simulink model "ExampleHeadTracking"  (Simulink 9.2)
settings: Solver=FixedStepDiscrete  StartTime=0.0  StopTime=inf  FixedStep=0.001  RelTol=1e-3  EnableMultiTasking=on
libraries: rFproPhysicsLib x3
settings Model: Creator=enewton  LastModifiedBy=SeanKavanagh
settings OptimizationCC: ExpressionDepthLimit=2147483647
settings DebuggingCC: SolverPrmCheckMsg=warning
settings RTWCC: SystemTargetFile=rfpro.tlc  MakeCommand="make_rtw OPTS=\"-DRUN_PHYSICS\""  TemplateMakefile=rfpro.tmf  Description=rFpro Target (Run Physics)  TargetLang=C++
settings STFCustomTargetCC: ModelReferenceCompliant=off  GeneratePreprocessorConditionals=Disable all  CombineOutputUpdateFcns=on  MatFileLogging=on  CPPClassGenCompliant=on  GRTInterface=off  SystemTargetFile=rfpro.tlc
settings GRTTargetCC: ModelReferenceCompliant=off  ParMdlRefBuildCompliant=off  CompOptLevelCompliant=off  ConcurrentExecutionCompliant=off  CombineOutputUpdateFcns=on  GRTInterface=off  UseToolchainInfoCompliant=off

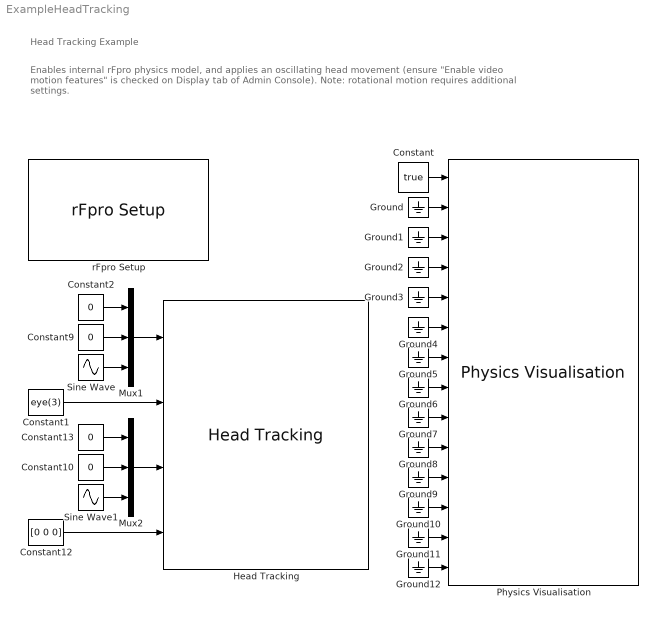
== system ExampleHeadTracking ==
  note: Enables internal rFpro physics model, and applies an oscillating head movement
      | (ensure "Enable video motion features" is checked on Display tab of Admin Console).
      |
      | Note: rotational motion requires additional settings.
  note: Head Tracking Example
  Constant : Constant  Value=true
  Constant1 : Constant  Value=eye(3)
  Constant{2,9..10,13} (4 alike) : Constant  Value=0
  Constant12 : Constant  Value=[0 0 0]
  Ground{,1..12} (13 alike) : Ground
  Head Tracking : rFproPhysicsLib/Head Tracking  period=-1  offset=0  useReverseByteOrder=off  rFpro__platform=Remote Model - Default
  Mux1 : Mux  Inputs=3
  Mux2 : Mux  Inputs=3
  Physics Visualisation : rFproPhysicsLib/Physics Visualisation  PAR_SKIP_INTERNAL_PHYSICS=off  PAR_ACCEL_VALID=off  PAR_ROT_ACCEL_VALID=off  PAR_GEAR_VALID=off  PAR_RPM_VALID=off  PAR_INPUTS_VALID=off  PAR_STEER_TORQUE_VALID=off  PAR_HEADLIGHTS_ON_VALID=off  PAR_WHEEL_POS_VALID=off  PAR_WHEEL_ORI_VALID=off  PAR_TYRE_PARAMS_VALID=off  PAR_WHEEL_ROTATION_VALID=off  PAR_WHEEL_BRAKE_TEMP_VALID=off  PAR_WHEEL_TREAD_TEMP_VALID=off  PAR_WHEEL_AIR_TEMP_VALID=off  period=-1  offset=0  useReverseByteOrder=on  rFpro__platform=Remote Model - Default
  Sine Wave : Sin  Frequency=2*pi / 1  SampleTime=0
  Sine Wave1 : Sin  Amplitude=1 * 2*pi / 1  Frequency=2*pi / 1  Phase=pi/2  SampleTime=0
  rFpro Setup : rFproPhysicsLib/rFpro Setup  platform=Remote Model - Default  stopOnSessionEnd=on  usePseudoRealtime=on  syncToRF=on  useReverseByteOrder=off  useRfTime=on  minIterations=4  maxIterations=1000  ipReceiveAddress='127.0.0.1'  ipReceivePort=11054  receiveSampleTime=-1  ipTransmitAddress='127.0.0.1'  ipTransmitPort=11052  transmitSampleTime=-1  pluginType=RUN_PHYSICS  sysTarget=xpctarget.tlc  templateMakeFile=xpc_default_tmf  makeCommand=make_rtw  buildDesc=xPC target
  wires:
  Constant/1 -> Physics Visualisation/1
  Ground/1 -> Physics Visualisation/2
  Ground1/1 -> Physics Visualisation/3
  Ground2/1 -> Physics Visualisation/4
  Ground3/1 -> Physics Visualisation/5
  Ground4/1 -> Physics Visualisation/6
  Ground5/1 -> Physics Visualisation/7
  Ground6/1 -> Physics Visualisation/8
  Ground7/1 -> Physics Visualisation/9
  Ground8/1 -> Physics Visualisation/10
  Ground9/1 -> Physics Visualisation/11
  Ground10/1 -> Physics Visualisation/12
  Ground11/1 -> Physics Visualisation/13
  Ground12/1 -> Physics Visualisation/14
  Constant2/1 -> Mux1/1
  Constant9/1 -> Mux1/2
  Sine Wave/1 -> Mux1/3
  Constant13/1 -> Mux2/1
  Constant10/1 -> Mux2/2
  Sine Wave1/1 -> Mux2/3
  Mux1/1 -> Head Tracking/1
  Mux2/1 -> Head Tracking/3
  Constant12/1 -> Head Tracking/4
  Constant1/1 -> Head Tracking/2
